simulink model "FindTarget"  (R2014a)
settings: Solver=FixedStepDiscrete  StartTime=0.0  StopTime=inf  RelTol=1e-3
undefined symbols (not defined in the file or in its folder): DiscIntNeverNeededParam
libraries: simulink x9, embdlinuxlib x3, visionstatistics x1, visiontextngfix x1
settings Model: SimulationMode=external  ExtModeTrigDuration=100  Creator=omcaree  LastModifiedBy=omcaree
settings OptimizationCC: OptimizeModelRefInitCode=on  LifeSpan=1
settings DebuggingCC: UnderspecifiedInitializationDetection=Classic  SolverPrmCheckMsg=none
settings HardwareCC: ProdLargestAtomicInteger=Long  ProdLargestAtomicFloat=Double  ProdEndianess=LittleEndian  ProdHWDeviceType=ARM Compatible->ARM Cortex
settings RTWCC: SystemTargetFile=realtime.tlc  GenerateMakefile=off  TemplateMakefile=realtime.tmf  Description=Run on Target Hardware  RTWVerbose=off  ProcessScript=realtime_make_rtw_hook  CustomSource=SerialPort.c
settings STFCustomTargetCC: TargetLibSuffix=.a  GenerateSampleERTMain=on  ConcurrentExecutionCompliant=off  GeneratePreprocessorConditionals=Use local settings  ERTCustomFileBanners=on  SupportNonInlinedSFcns=off  SupportVariableSizeSignals=on  MATLABClassNameForMDSCustomization=Simulink.SoftwareTarget.ERTCustomization  GRTInterface=off  SystemTargetFile=realtime.tlc
settings ERTTargetCC: CombineOutputUpdateFcns=off  SupportContinuousTime=on  SupportVariableSizeSignals=on  ExtModeMexArgs='192.168.0.1' 0 17725  ERTSrcFileBannerTemplate=realtime_code_template.cgt  ERTHdrFileBannerTemplate=realtime_code_template.cgt  ERTDataSrcFileTemplate=realtime_code_template.cgt  ERTDataHdrFileTemplate=realtime_code_template.cgt  ERTCustomFileTemplate=realtime_file_process.tlc

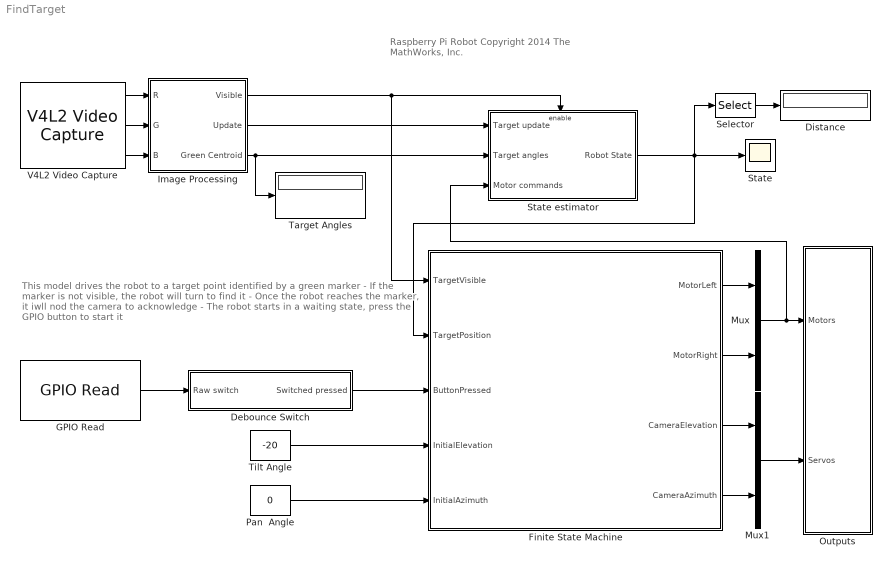
== system FindTarget ==
  note: Raspberry Pi Robot
      | Copyright 2014 The MathWorks, Inc.
  note: This model drives the robot to a target point identified by a green marker
      |  - If the marker is not visible, the robot will turn to find it
      |  - Once the robot reaches the marker, it iwll nod the camera to acknowledge
      |  - The robot starts in a waiting state, press the GPIO button to start it
  Debounce Switch : Subsystem
  Distance : Display
  Finite State Machine : Stateflow chart  TreatAsAtomicUnit=on
  GPIO Read : embdlinuxlib/GPIO Read  board=Model B Rev2  gpio=18  internalResistor=Off  sampleTime=1/30  direction=Input  blockPlatform=Raspberry Pi
  Image Processing : Subsystem
  Mux : Mux  Inputs=2
  Mux1 : Mux  Inputs=2
  Outputs : Subsystem
  Pan  Angle : Constant  Value=0
  Selector : Selector  InputPortWidth=3
  State : Scope
      settings: YMin=-0.45  YMax=0.25
  State estimator : Subsystem
  Target Angles : Display
  Tilt Angle : Constant  Value=-20
  V4L2 Video Capture : embdlinuxlib/V4L2 Video Capture  m_devName='/dev/video0'  roi=[0, 0, 640, 480]  imSizeSelection=320x240  imSize=[160 128]  pixelFormat=RGB  pixelOrder=Planar  sampleTime=1/30  simOutput=Colorbars  blockPlatform=Raspberry Pi
  wires:
  Image Processing/3(Green Centroid) -> Target Angles/1, State estimator/2(Target angles)
  Image Processing/2(Update) -> State estimator/1(Target update)
  State estimator/1(Robot State) -> Selector/1, State/1, Finite State Machine/2(TargetPosition)
  V4L2 Video Capture/1 -> Image Processing/1(R)
  V4L2 Video Capture/2 -> Image Processing/2(G)
  V4L2 Video Capture/3 -> Image Processing/3(B)
  Mux/1 -> Outputs/1(Motors), State estimator/3(Motor commands)
  Finite State Machine/2(MotorRight) -> Mux/2
  Finite State Machine/1(MotorLeft) -> Mux/1
  Image Processing/1(Visible) -> State estimator/Enable, Finite State Machine/1(TargetVisible)
  GPIO Read/1 -> Debounce Switch/1(Raw switch)
  Debounce Switch/1(Switched pressed) -> Finite State Machine/3(ButtonPressed)
  Mux1/1 -> Outputs/2(Servos)
  Tilt Angle/1 -> Finite State Machine/4(InitialElevation)
  Pan  Angle/1 -> Finite State Machine/5(InitialAzimuth)
  Finite State Machine/3(CameraElevation) -> Mux1/1
  Finite State Machine/4(CameraAzimuth) -> Mux1/2
  Selector/1 -> Distance/1

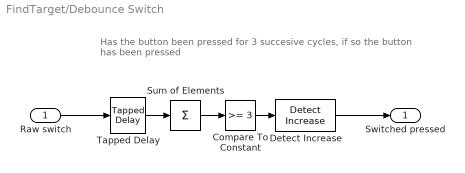
== system FindTarget/Debounce Switch ==
  note: Has the button been pressed for 3 succesive cycles, if so the
      | button has been pressed
  Raw switch : Inport
  Compare To Constant : simulink/Logic and Bit Operations/Compare To Constant  relop=>=  const=3  OutDataTypeStr=boolean
  Detect Increase : simulink/Logic and Bit Operations/Detect Increase  vinit=0.0  InputProcessing=Inherited  OutDataTypeStr=boolean
  Sum of Elements : Sum  Inputs=+
  Tapped Delay : simulink/Discrete/Tapped Delay  vinit=0.0  samptime=-1  NumDelays=3  DelayOrder=Oldest  includeCurrent=off
  Switched pressed : Outport
  wires:
  Raw switch/1 -> Tapped Delay/1
  Tapped Delay/1 -> Sum of Elements/1
  Sum of Elements/1 -> Compare To Constant/1
  Compare To Constant/1 -> Detect Increase/1
  Detect Increase/1 -> Switched pressed/1

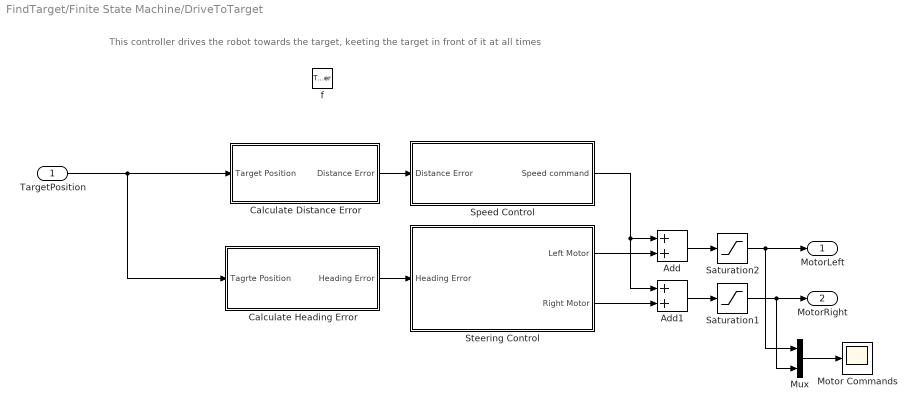
== system FindTarget/Finite State Machine/DriveToTarget ==
  note: This controller drives the robot towards the target, keeting the target in front of it at all times
  TargetPosition : Inport  OutDataTypeStr=double  PortDimensions=3
  f : TriggerPort  TriggerType=function-call  StatesWhenEnabling=reset  SampleTimeType=periodic  SampleTime=1/30
      settings: CopyFcn=Stateflow.SLINSF.SimulinkMan.removeBlockPreDeleteFcn  PreDeleteFcn=Stateflow.SLINSF.SimulinkMan.unsafePredeleteFcn
  Add : Sum
  Add1 : Sum
  Calculate Distance Error : Subsystem
  Calculate Heading Error : Subsystem
  Motor Commands : Scope
      settings: SaveName=ScopeData2
  Mux : Mux  Inputs=2
  Saturation1 : Saturate  UpperLimit=30  LowerLimit=-30
  Saturation2 : Saturate  UpperLimit=30  LowerLimit=-30
  Speed Control : Subsystem
  Steering Control : Subsystem
  MotorLeft : Outport  PortDimensions=1
  MotorRight : Outport  Port=2  PortDimensions=1
  wires:
  Steering Control/1(Left Motor) -> Add/2
  Steering Control/2(Right Motor) -> Add1/2
  Add1/1 -> Saturation1/1
  Add/1 -> Saturation2/1
  Saturation1/1 -> Mux/2, MotorRight/1
  TargetPosition/1 -> Calculate Heading Error/1(Tagrte Position), Calculate Distance Error/1(Target Position)
  Speed Control/1(Speed command) -> Add1/1, Add/1
  Calculate Heading Error/1(Heading Error) -> Steering Control/1(Heading Error)
  Calculate Distance Error/1(Distance Error) -> Speed Control/1(Distance Error)
  Mux/1 -> Motor Commands/1
  Saturation2/1 -> Mux/1, MotorLeft/1

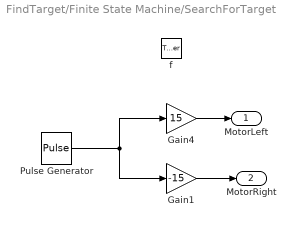
== system FindTarget/Finite State Machine/SearchForTarget ==
  f : TriggerPort  TriggerType=function-call  StatesWhenEnabling=reset  SampleTimeType=periodic  SampleTime=1/30
      settings: CopyFcn=Stateflow.SLINSF.SimulinkMan.removeBlockPreDeleteFcn  PreDeleteFcn=Stateflow.SLINSF.SimulinkMan.unsafePredeleteFcn
  Gain1 : Gain  Gain=-15
  Gain4 : Gain  Gain=15
  Pulse Generator : DiscretePulseGenerator  Period=10  PulseWidth=5  SampleTime=-1
  MotorLeft : Outport  OutDataTypeStr=double
  MotorRight : Outport  Port=2  OutDataTypeStr=double
  wires:
  Gain1/1 -> MotorRight/1
  Gain4/1 -> MotorLeft/1
  Pulse Generator/1 -> Gain1/1, Gain4/1

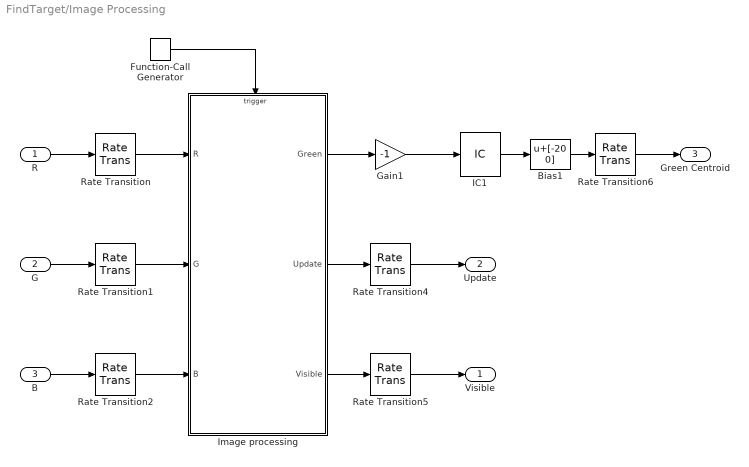
== system FindTarget/Image Processing ==
  R : Inport
  G : Inport  Port=2
  B : Inport  Port=3
  Bias1 : Bias  Bias=[-20 0]
  Function-Call Generator : simulink/Ports & Subsystems/Function-Call Generator  sample_time=1/3  numberOfIterations=1
  Gain1 : Gain  Gain=-1
  IC1 : InitialCondition  Value=[-20 0]
  Image processing : Subsystem
  Rate Transition{,1..2,4..6} (6 alike) : RateTransition
  Visible : Outport
  Update : Outport  Port=2
  Green Centroid : Outport  Port=3
  wires:
  G/1 -> Rate Transition1/1
  B/1 -> Rate Transition2/1
  R/1 -> Rate Transition/1
  Function-Call Generator/1 -> Image processing/Trigger
  Image processing/2(Update) -> Rate Transition4/1
  Rate Transition1/1 -> Image processing/2(G)
  Rate Transition/1 -> Image processing/1(R)
  Rate Transition2/1 -> Image processing/3(B)
  Image processing/3(Visible) -> Rate Transition5/1
  Rate Transition5/1 -> Visible/1
  Rate Transition4/1 -> Update/1
  Gain1/1 -> IC1/1
  Image processing/1(Green) -> Gain1/1
  IC1/1 -> Bias1/1
  Rate Transition6/1 -> Green Centroid/1
  Bias1/1 -> Rate Transition6/1

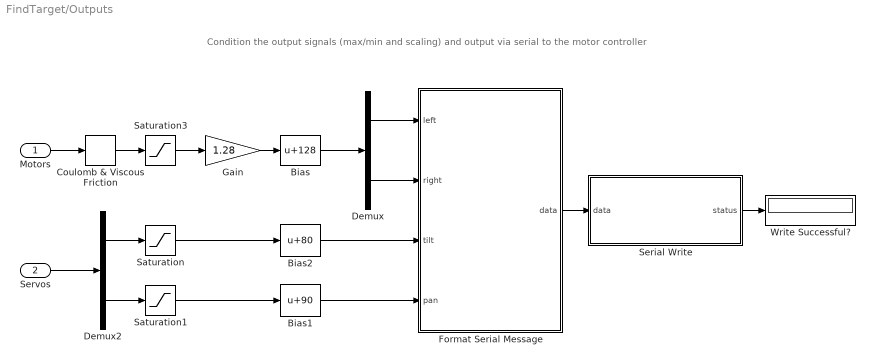
== system FindTarget/Outputs ==
  note: Condition the output signals (max/min and scaling) and output via serial to the motor controller
  Motors : Inport
  Servos : Inport  Port=2
  Bias : Bias  Bias=128
  Bias1 : Bias  Bias=90
  Bias2 : Bias  Bias=80
  Coulomb & Viscous Friction : simulink/Discontinuities/Coulomb & Viscous Friction  offset=5  gain=1
  Demux : Demux  Outputs=2
  Demux2 : Demux  Outputs=2
  Format Serial Message : MATLAB Function  TreatAsAtomicUnit=on
  Gain : Gain  Gain=1.28
  Saturation : Saturate  UpperLimit=10  LowerLimit=-30
  Saturation1 : Saturate  UpperLimit=10  LowerLimit=-30
  Saturation3 : Saturate  UpperLimit=100  LowerLimit=-100
  Serial Write : MATLAB Function  TreatAsAtomicUnit=on
  Write Successful? : Display
  wires:
  Motors/1 -> Coulomb & Viscous Friction/1
  Format Serial Message/1(data) -> Serial Write/1(data)
  Saturation3/1 -> Gain/1
  Gain/1 -> Bias/1
  Bias/1 -> Demux/1
  Demux/2 -> Format Serial Message/2(right)
  Coulomb & Viscous Friction/1 -> Saturation3/1
  Demux/1 -> Format Serial Message/1(left)
  Demux2/1 -> Saturation/1
  Servos/1 -> Demux2/1
  Demux2/2 -> Saturation1/1
  Bias2/1 -> Format Serial Message/3(tilt)
  Saturation/1 -> Bias2/1
  Saturation1/1 -> Bias1/1
  Bias1/1 -> Format Serial Message/4(pan)
  Serial Write/1(status) -> Write Successful?/1

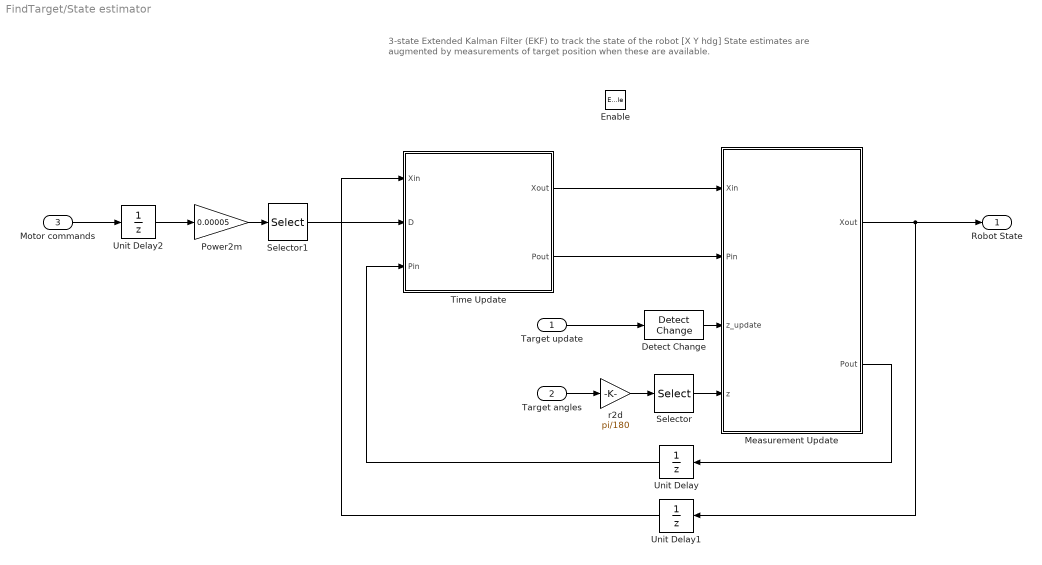
== system FindTarget/State estimator ==
  note: 3-state Extended Kalman Filter (EKF) to track the state of the robot [X Y hdg]
      |
      | State estimates are augmented by measurements of target position when these are available.
  Target update : Inport
  Target angles : Inport  Port=2
  Motor commands : Inport  Port=3
  Enable : EnablePort  StatesWhenEnabling=reset
  Detect Change : simulink/Logic and Bit Operations/Detect Change  vinit=0  InputProcessing=Inherited  OutDataTypeStr=boolean
  Measurement Update : MATLAB Function  TreatAsAtomicUnit=on
  Power2m : Gain  Gain=0.00005
  Selector : Selector  InputPortWidth=2  Indices=[2 1]
  Selector1 : Selector  InputPortWidth=2  Indices=[2 1]
  Time Update : MATLAB Function  TreatAsAtomicUnit=on
  Unit Delay : UnitDelay  InitialCondition=0.1*eye(3)  SampleTime=-1
  Unit Delay1 : UnitDelay  InitialCondition=[-0.4 0 0]'  SampleTime=-1
  Unit Delay2 : UnitDelay  InitialCondition=[0 0]  SampleTime=-1
  r2d : Gain  Gain=pi/180
  Robot State : Outport
  wires:
  Measurement Update/1(Xout) -> Robot State/1, Unit Delay1/1
  Target angles/1 -> r2d/1
  Motor commands/1 -> Unit Delay2/1
  Unit Delay/1 -> Time Update/3(Pin)
  Time Update/2(Pout) -> Measurement Update/2(Pin)
  Time Update/1(Xout) -> Measurement Update/1(Xin)
  Measurement Update/2(Pout) -> Unit Delay/1
  Target update/1 -> Detect Change/1
  Power2m/1 -> Selector1/1
  Unit Delay1/1 -> Time Update/1(Xin)
  Selector/1 -> Measurement Update/4(z)
  r2d/1 -> Selector/1
  Selector1/1 -> Time Update/2(D)
  Unit Delay2/1 -> Power2m/1
  Detect Change/1 -> Measurement Update/3(z_update)

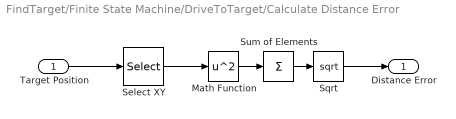
== system FindTarget/Finite State Machine/DriveToTarget/Calculate Distance Error ==
  Target Position : Inport
  Math Function : Math  Operator=square  SaturateOnIntegerOverflow=on
  Select XY : Selector  InputPortWidth=3  Indices=[1 2]
  Sqrt : Sqrt  SaturateOnIntegerOverflow=on
  Sum of Elements : Sum  Inputs=+
  Distance Error : Outport
  wires:
  Select XY/1 -> Math Function/1
  Math Function/1 -> Sum of Elements/1
  Sum of Elements/1 -> Sqrt/1
  Sqrt/1 -> Distance Error/1
  Target Position/1 -> Select XY/1

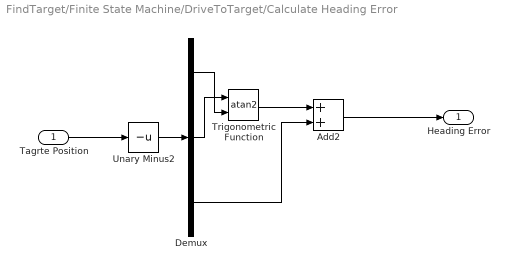
== system FindTarget/Finite State Machine/DriveToTarget/Calculate Heading Error ==
  Tagrte Position : Inport
  Add2 : Sum
  Demux : Demux  Outputs=3
  Trigonometric Function : Trigonometry  Operator=atan2
  Unary Minus2 : UnaryMinus
  Heading Error : Outport
  wires:
  Demux/2 -> Trigonometric Function/1
  Demux/1 -> Trigonometric Function/2
  Add2/1 -> Heading Error/1
  Trigonometric Function/1 -> Add2/1
  Demux/3 -> Add2/2
  Unary Minus2/1 -> Demux/1
  Tagrte Position/1 -> Unary Minus2/1

== system FindTarget/Finite State Machine/DriveToTarget/Speed Control ==
  Distance Error : Inport
  Saturation3 : Saturate  UpperLimit=10  LowerLimit=0
  Speed Gain : Gain  Gain=45
  Speed command : Outport
  wires:
  Speed Gain/1 -> Saturation3/1
  Saturation3/1 -> Speed command/1
  Distance Error/1 -> Speed Gain/1

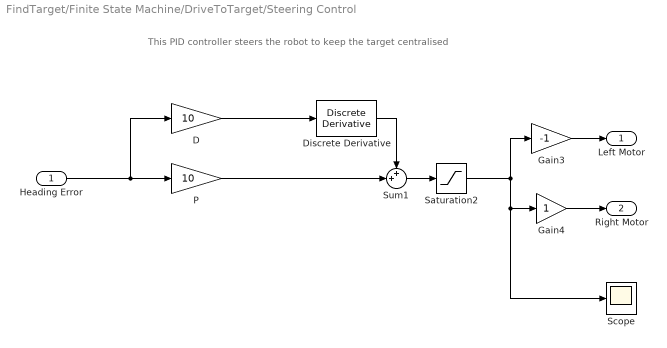
== system FindTarget/Finite State Machine/DriveToTarget/Steering Control ==
  note: This PID controller steers the robot to keep the target centralised
  Heading Error : Inport  OutDataTypeStr=double  PortDimensions=1
  D : Gain  Gain=10
  Discrete Derivative : simulink/Discrete/Discrete Derivative  gainval=1.0  ICPrevScaledInput=0.0  InputProcessing=Inherited  OutMin=[]  OutMax=[]  OutDataType=fixdt(1, 16)  OutScaling=2^-10  DoSatur=off
  Gain3 : Gain  Gain=-1
  Gain4 : Gain
  P : Gain  Gain=10
  Saturation2 : Saturate  UpperLimit=20  LowerLimit=-20
  Scope : Scope
  Sum1 : Sum  Inputs=++|
  Left Motor : Outport
  Right Motor : Outport  Port=2
  wires:
  Gain3/1 -> Left Motor/1
  Gain4/1 -> Right Motor/1
  Sum1/1 -> Saturation2/1
  P/1 -> Sum1/2
  Discrete Derivative/1 -> Sum1/1
  D/1 -> Discrete Derivative/1
  Saturation2/1 -> Gain3/1, Scope/1, Gain4/1
  Heading Error/1 -> D/1, P/1

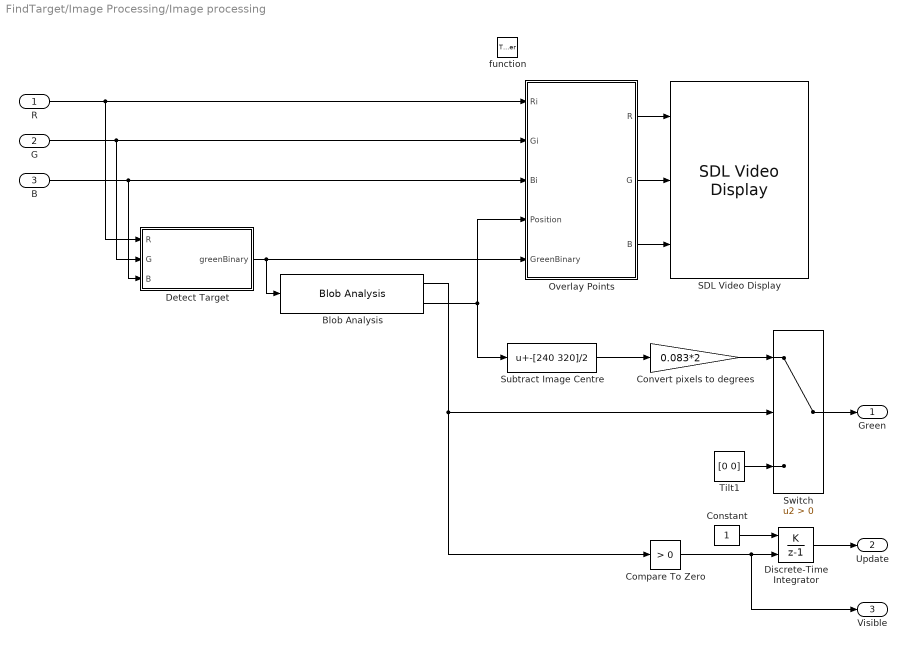
== system FindTarget/Image Processing/Image processing ==
  R : Inport
  G : Inport  Port=2
  B : Inport  Port=3
  function : TriggerPort  TriggerType=function-call  StatesWhenEnabling=reset
  Blob Analysis : visionstatistics/Blob Analysis  Tag=vipblks_row_conv  area=on  centroid=on  bBox=off  majorAxis=off  minorAxis=off  angle=off  eccentricity=off  equivDiameterSq=off  extent=off  perimeter=off  maxBlobs=1  warnIfNumBlobsExceeded=off  isCount=off  useMinArea=on  minArea=100  useMaxArea=off  maxArea=intmax('uint32')  excludeBorderBlob=off  outDT=double  isOutVarDim=off  isFill=on  fillValues=-1  conn=8  isLabel=off  outputMode=Binary point scaling  outputWordLength=32  outputFracLength=16  firstCoeffMode=Binary point scaling  firstCoeffWordLength=16  firstCoeffFracLength=14  secondCoeffMode=Binary point scaling  secondCoeffWordLength=32  secondCoeffFracLength=16  accumMode=Binary point scaling  accumWordLength=32  accumFracLength=0  prodOutputMode=Binary point scaling  prodOutputWordLength=32  prodOutputFracLength=16  roundingMode=Floor  overflowMode=off
  Compare To Zero : simulink/Logic and Bit Operations/Compare To Zero  relop=>  OutDataTypeStr=boolean
  Constant : Constant
  Convert pixels to degrees : Gain  Gain=0.083*2
  Detect Target : Subsystem
  Discrete-Time Integrator : DiscreteIntegrator  IntegratorMethod=Accumulation: Forward Euler  ExternalReset=rising  SampleTime=-1  ICPrevOutput=DiscIntNeverNeededParam  ICPrevScaledInput=DiscIntNeverNeededParam
  Overlay Points : Subsystem
  SDL Video Display : embdlinuxlib/SDL Video Display  pixelFormat=RGB  pixelOrder=Planar  rowMajor=on  blockPlatform=Raspberry Pi
  Subtract Image Centre : Bias  Bias=-[240 320]/2
  Switch : Switch  Criteria=u2 > Threshold
  Tilt1 : Constant  Value=[0 0]
  Green : Outport
  Update : Outport  Port=2
  Visible : Outport  Port=3
  wires:
  Detect Target/1(greenBinary) -> Overlay Points/5(GreenBinary), Blob Analysis/1
  G/1 -> Detect Target/2(G), Overlay Points/2(Gi)
  R/1 -> Detect Target/1(R), Overlay Points/1(Ri)
  Blob Analysis/1 -> Switch/2, Compare To Zero/1
  Blob Analysis/2 -> Overlay Points/4(Position), Subtract Image Centre/1
  B/1 -> Detect Target/3(B), Overlay Points/3(Bi)
  Convert pixels to degrees/1 -> Switch/1
  Subtract Image Centre/1 -> Convert pixels to degrees/1
  Tilt1/1 -> Switch/3
  Switch/1 -> Green/1
  Compare To Zero/1 -> Visible/1, Discrete-Time Integrator/2
  Constant/1 -> Discrete-Time Integrator/1
  Discrete-Time Integrator/1 -> Update/1
  Overlay Points/2(G) -> SDL Video Display/2
  Overlay Points/3(B) -> SDL Video Display/3
  Overlay Points/1(R) -> SDL Video Display/1

== system FindTarget/Image Processing/Image processing/Detect Target ==
  note: Calculate the green intensity and binary images using the same process as in MATLAB
  R : Inport
  G : Inport  Port=2
  B : Inport  Port=3
  Calculate Green Intensity : MATLAB Function  TreatAsAtomicUnit=on
  Compare To Threshold : simulink/Logic and Bit Operations/Compare To Constant  relop=>  const=40  OutDataTypeStr=boolean
  greenBinary : Outport
  wires:
  B/1 -> Calculate Green Intensity/3(blue)
  R/1 -> Calculate Green Intensity/1(red)
  G/1 -> Calculate Green Intensity/2(green)
  Compare To Threshold/1 -> greenBinary/1
  Calculate Green Intensity/1(greenIntensity) -> Compare To Threshold/1

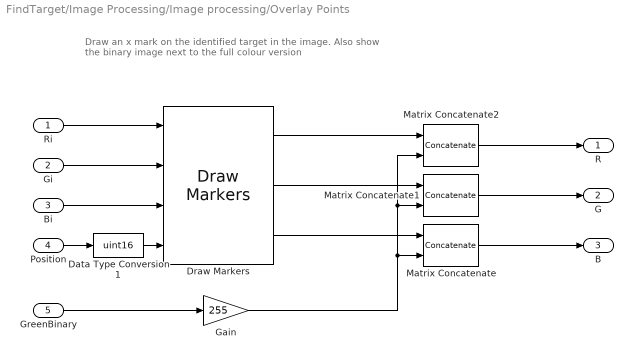
== system FindTarget/Image Processing/Image processing/Overlay Points ==
  note: Draw an x mark on the identified target in the image.
      | Also show the binary image next to the full colour version
  Ri : Inport
  Gi : Inport  Port=2
  Bi : Inport  Port=3
  Position : Inport  Port=4
  GreenBinary : Inport  Port=5
  Data Type Conversion1 : DataTypeConversion  OutDataTypeStr=uint16
  Draw Markers : visiontextngfix/Draw Markers  shape=X-mark  size=5  fill=off  fillClrSource=Specify via dialog  display=User-specified value  intensity=200  color=[255 0 0]  opacity=0.6  viewport=Entire image  antialiasing=off  inType=Obsolete  imagePorts=Separate color signals  prodOutputMode=Binary point scaling  prodOutputWordLength=32  prodOutputFracLength=14  memoryMode=Specify word length  memoryWordLength=16  memoryFracLength=15  roundingMode=Floor  overflowMode=off
  Gain : Gain  Gain=255  OutDataTypeStr=uint8
  Matrix Concatenate : Concatenate  Mode=Multidimensional array
  Matrix Concatenate1 : Concatenate  Mode=Multidimensional array
  Matrix Concatenate2 : Concatenate  Mode=Multidimensional array
  R : Outport
  G : Outport  Port=2
  B : Outport  Port=3
  wires:
  Draw Markers/2 -> Matrix Concatenate1/1
  Draw Markers/3 -> Matrix Concatenate/1
  Draw Markers/1 -> Matrix Concatenate2/1
  Data Type Conversion1/1 -> Draw Markers/4
  Position/1 -> Data Type Conversion1/1
  Bi/1 -> Draw Markers/3
  Gi/1 -> Draw Markers/2
  Ri/1 -> Draw Markers/1
  GreenBinary/1 -> Gain/1
  Gain/1 -> Matrix Concatenate2/2, Matrix Concatenate1/2, Matrix Concatenate/2
  Matrix Concatenate/1 -> B/1
  Matrix Concatenate2/1 -> R/1
  Matrix Concatenate1/1 -> G/1

== matlab function FindTarget/State estimator/Measurement Update ==
  data: Xin input; Pin input; z_update input; Xout output; z input; Pout output
function [Xout, Pout] = MeasurementUpdate(Xin,Pin,z_update,z)
%#codegen

% Only perform measurement update if we have a new measurement
if (z_update)
    % Initialise some parameters
    targetX = [0 0]';
    height = 0.14;
    d = sqrt(sum((targetX - Xin(1:2)).^2));
    H = zeros(2,3);

    % Calculate measurement matrix
    H(1,1) = (targetX(2) - Xin(2)) / d^2;
    H(1,2) = (-targetX(1) + Xin(1)) / d^2;
    H(1,3) = -1;
    H(2,1) = -height*(targetX(1) - Xin(1))/ (d * (height^2 + d^2));
    H(2,2) = -height*(targetX(2) - Xin(2))/ (d * (height^2 + d^2));
    H(2,3) = 0;

    % Calculate Kalman gain
    R = 0.05*eye(2);
    K = Pin*H'*(H*Pin*H'+R)^(-1);

    % Calculate predicted measurements
    h = zeros(2,1);
    h(1) = atan2((targetX(2) - Xin(2)),(targetX(1) - Xin(1))) - Xin(3);
    h(2) = -atan2(height,d);

    % Update state
    Xout = Xin + K*(z-h);

    % Update covariance
    Pout = (eye(3) - K*H)*Pin*(eye(3)-K*H)' + K*R*K';
else
    Xout = Xin;
    Pout = Pin;
end

== matlab function FindTarget/Image Processing/Image processing/Detect Target/Calculate Green Intensity ==
  data: red input; greenIntensity output; green input; blue input
function greenIntensity = calculateGreenIntensity(red, green, blue)

greenIntensity = green - red/2 - blue/2;

== matlab function FindTarget/Outputs/Format Serial Message ==
  settings: fimath=|
      | fimath('RoundingMethod', 'Floor', ...
      |     'OverflowAction', 'Wrap', ...
      |     'ProductMode', 'FullPrecision', ...
      |     'SumMode', 'FullPrecision')
  data: left input; right input; tilt input; data output; pan input
function data = formatMotorMessage(left, right, tilt, pan)
%#codegen

messageID = uint8(2);   % Command
messageLength = uint8(9);

data = uint8([255 255 messageID messageLength uint8(left) uint8(right) uint8(pan) uint8(tilt) 0]');

% Checksum is the complement of the sum of each byte
% Excluding start characters
sum = uint32(0);
for i=3:(messageLength-1)
    sum = sum + uint32(data(i));
end

data(end) = uint8(bitcmp(sum,'uint32'));

== matlab function FindTarget/Outputs/Serial Write ==
  data: data input; status output
function status = SerialWrite(data)
%#codegen
persistent spHandle;
status = false;
if ~coder.target('SFun')
    if isempty(spHandle) 
        spHandle = int32(0);
        spHandle = coder.ceval('setupSerialPort',['/dev/ttyAMA0' 0],uint32(57600));
    end
    if (spHandle > 0)
        bytesTransmitted = int32(0);
        bytesTransmitted = coder.ceval('write',spHandle,coder.ref(data),uint32(length(data)));
        if bytesTransmitted == length(data)
            status = true;
        end
    end
end

== matlab function FindTarget/State estimator/Time Update ==
  data: Xin input; Xout output; D input; Pin input; Pout output
function [Xout, Pout] = TimeUpdate(Xin,D,Pin)
%#codegen

% calculate some initial parameters
b = 0.1;
delD = sum(D)/2;
delPhi = (D(1) - D(2)) / b;
Q = 0.001*eye(3);

% Update state
Xout = Xin + [delD*cos(Xin(3) + delPhi/2); delD*sin(Xin(3) + delPhi/2); delPhi];

% Calculate A-matrix
A = eye(3,3);
A(1,3) = -delD*sin(Xout(3) + delPhi/2);
A(2,3) = delD*cos(Xout(3) + delPhi/2);

% Calculate B-matrix
B = eye(3,2);
B(1,1) = cos(Xout(3) + delPhi/2)/2 + delD*sin(Xout(3) + delPhi/2)/2/b;
B(1,2) = cos(Xout(3) + delPhi/2)/2 - delD*sin(Xout(3) + delPhi/2)/2/b;
B(2,1) = sin(Xout(3) + delPhi/2)/2 - delD*cos(Xout(3) + delPhi/2)/2/b;
B(2,2) = sin(Xout(3) + delPhi/2)/2 + delD*cos(Xout(3) + delPhi/2)/2/b;
B(3,1) = -1/b;
B(3,2) = 1/b;

% Update covariance matrix
Pout = A*Pin*A' + 0.01^2*(B*B') + Q;

== stateflow chart FindTarget/Finite State Machine ==
  state Start
    entry: MotorLeft = 0;
    entry: MotorRight = 0;
    entry: CameraElevation = InitialElevation
    entry: CameraAzimuth = InitialAzimuth
  state Waiting
  state Running
    state Search
      during: [MotorLeft,MotorRight] = SearchForTarget
    state Drive
      during: [MotorLeft,MotorRight] = DriveToTarget(TargetPosition)
    state Nod
      entry: i = 0;
      exit: CameraElevation = 0;
      state Up
        entry: CameraElevation = 10;
        entry: i = i + 1;
      state Down
        entry: CameraElevation = -30;
        entry: i = i + 1;
      Up -> Down : after(200,msec)
      Down -> Up : after(200,msec)
    state Stop
      entry: MotorLeft = 0;
      entry: MotorRight= 0;
    Search -> Drive : [TargetVisible]
    Drive -> Stop : [~TargetVisible]
    Stop -> Up
  state [MotorLeft,MotorRight] = DriveToTarget(TargetPosition) [function]
  state [MotorLeft,MotorRight] = SearchForTarget [function]
  (default) -> Start
  Nod -> Start : [i>10]
  Running -> Start : [ButtonPressed]
  Start -> Waiting : after(1,sec)
  Waiting -> Search : [ButtonPressed]
  data: MotorLeft function_output size=1; MotorRight function_output size=1; TargetPosition function_input double size=3; MotorLeft function_output double; MotorRight function_output double; TargetVisible input; TargetPosition input; MotorLeft output; MotorRight output; ButtonPressed input; i local; InitialElevation input; InitialAzimuth input; CameraElevation output; CameraAzimuth output
